simulink model "CompFeatures_testHarness"  (R2012b)
settings: Solver=FixedStepDiscrete  StartTime=0.0  StopTime=50  RelTol=1e-3
InitFcn:
  | N=256;
  | Fs = 1000;
  | bw = 5.6;
undefined symbols (not defined in the file): sigbuilder_block
libraries: simulink x4, ResultLoggerLib x3
settings Model: RequirementInfo={'other' '..\..\..\..\requirements\ebd_srs.doc' '@Simulink_requirement_item_4' 'true' 'Filter input signal via polyphase digital filter bank' 'Requirement' } %GIDa_bfa4a348_cd9f_4101_a776_3ea215f34dae  SldvGeneratedHarnessModel=TestUnitModel=CompFeatures|  RecordCoverage=on  CovMetricSettings=dcmtroie  CovHTMLOptions=-sRT=1 -aTS=1 -bRG=1 -bTC=0 -hTR=0 -nFC=0 -scm=1 -bcm=1 -xEv=0  CovExternalEMLEnable=on  Creator=aanantha  LastModifiedBy=klindqvi
settings DataIOCC: SaveFormat=Structure  SignalLoggingSaveFormat=ModelDataLogs  SaveOutput=off  SaveTime=off  SignalLoggingName=logsOut
settings OptimizationCC: InlineParams=on  OptimizeModelRefInitCode=on  LifeSpan=1
settings DebuggingCC: ReadBeforeWriteMsg=DisableAll  WriteAfterWriteMsg=DisableAll  WriteAfterReadMsg=DisableAll  SolverPrmCheckMsg=none  InheritedTsInSrcMsg=none  ParameterPrecisionLossMsg=none  FcnCallInpInsideContextMsg=EnableAllAsWarning  ModelReferenceSymbolNameMessage=none
settings HardwareCC: ProdLargestAtomicInteger=Long  ProdLargestAtomicFloat=Double  ProdEndianess=LittleEndian  ProdHWDeviceType=ARM Compatible->ARM Cortex
settings ModelReferenceCC: UpdateModelReferenceTargets=AssumeUpToDate  CheckModelReferenceTargetMessage=none
settings RTWCC: SystemTargetFile=ert.tlc  TemplateMakefile=ert_default_tmf  Description=Embedded Coder  GenerateReport=on  ProcessScript=ert_make_rtw_hook  IncludeHyperlinkInReport=on  LaunchReport=on  GenerateTraceInfo=on  GenerateTraceReportSl=on  GenerateTraceReportSf=on  GenerateTraceReportEml=on  GenerateCodeMetricsReport=on
settings CodeAppCC: IgnoreCustomStorageClasses=off
settings ERTTargetCC: CodeReplacementLibrary=GCC ARM Cortex-A8  MultiwordLength=2048  GenerateSampleERTMain=on  ERTCustomFileTemplate=example_file_process.tlc  ConvertIfToSwitch=off  SuppressUnreachableDefaultCases=off

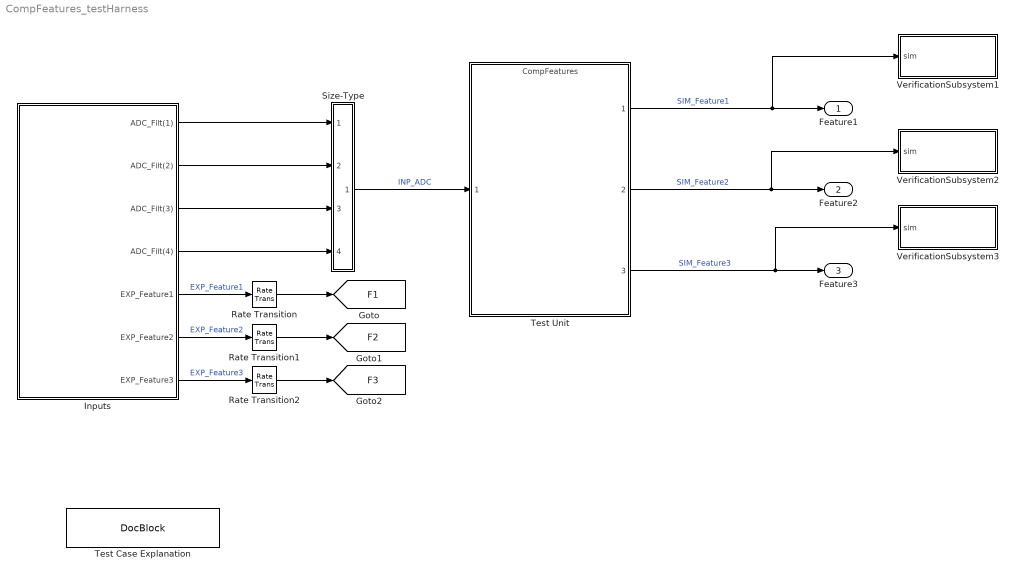
== system CompFeatures_testHarness ==
  Inputs : Subsystem  Tag=STV Subsys  RequirementInfo={'other' '..\..\..\..\requirements\ebd_srs.doc' '@REQ001- Filter input signal via polyphase digital filter bank' 'true' 'REQ001- Filter input signal via polyphase digital filter bank' '' } %GIDa_c0a67702_d4ee_4461_aee3_06328e90f161  LoadFcn=sigbuilder_block('load');  StartFcn=sigbuilder_block('start');  StopFcn=sigbuilder_block('stop');  ClipboardFcn=sigbuilder_block('clipboard');  mask(Sigbuilder block){}
      mask init:
      | if ~strcmp(get_param(bdroot(gcb),'SimulationStatus'),'stopped'),tuvar = sigbuilder_block('maskInit'); end
      settings: CopyFcn=sigbuilder_block('copy');  DeleteFcn=sigbuilder_block('delete');  ModelCloseFcn=sigbuilder_block('modelClose');  PreSaveFcn=sigbuilder_block('preSave');  PauseFcn=sigbuilder_block('pause');  ContinueFcn=sigbuilder_block('continue');  NameChangeFcn=sigbuilder_block('namechange');  OpenFcn=sigbuilder_block('open',[49.5 50.25 519.75 603 ]);  CloseFcn=sigbuilder_block('close');
      mask Display: plot(0, 0, 100, 100,[2, 2, 32, 32, 2], [68, 8, 8, 68, 68],[32, 2], [38, 38], [32, 19, 2],[53, 60, 44], [32, 17, 17, 2],[16, 16, 31, 31]);txt = getActiveGroup(gcbh);text(2, 100, txt,'verticalAlignment', 'top');
  Rate Transition : RateTransition  Integrity=off
  Rate Transition1 : RateTransition  Integrity=off
  Rate Transition2 : RateTransition  Integrity=off
  Size-Type : Subsystem
  Test Case Explanation : simulink/Model-Wide Utilities/DocBlock  DocumentType=Text
      content=|
      | Test case with default values because no SLDVDATA supplied
  Test Unit : ModelReference  ModelNameDialog=CompFeatures  SimulationMode=Normal  ModelReferenceVersion=1.280  CopyOfModelName=CompFeatures  DefaultDataLogging=on
  VerificationSubsystem1 : Subsystem
  VerificationSubsystem2 : Subsystem
  VerificationSubsystem3 : Subsystem
  Feature1 : Outport  OutDataTypeStr=single  PortDimensions=1  SampleTime=[0.08900000000000001,0]
  Feature2 : Outport  Port=2  OutDataTypeStr=single  PortDimensions=1  SampleTime=[0.08900000000000001,0]
  Feature3 : Outport  Port=3  OutDataTypeStr=single  PortDimensions=1  SampleTime=[0.08900000000000001,0]
  tag scope: F1=global, F2=global, F3=global
  wires:
  Size-Type/1(Out1) -> Test Unit/1  "INP_ADC"
  Test Unit/1 -> VerificationSubsystem1/1("sim "), Feature1/1  "SIM_Feature1"
  Test Unit/2 -> VerificationSubsystem2/1("sim "), Feature2/1  "SIM_Feature2"
  Test Unit/3 -> VerificationSubsystem3/1("sim "), Feature3/1  "SIM_Feature3"
  Inputs/5(EXP_Feature1) -> Rate Transition/1  "EXP_Feature1"
  Inputs/7(EXP_Feature3) -> Rate Transition2/1  "EXP_Feature3"
  Inputs/6(EXP_Feature2) -> Rate Transition1/1  "EXP_Feature2"
  Inputs/1(ADC_Filt(1)) -> Size-Type/1(In1)
  Inputs/2(ADC_Filt(2)) -> Size-Type/2(In2)
  Inputs/3(ADC_Filt(3)) -> Size-Type/3(In3)
  Inputs/4(ADC_Filt(4)) -> Size-Type/4(In4)
  Rate Transition/1 -> [F1]
  Rate Transition1/1 -> [F2]
  Rate Transition2/1 -> [F3]

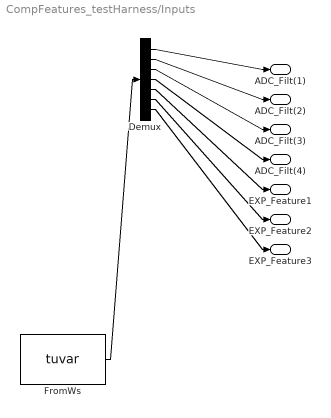
== system CompFeatures_testHarness/Inputs ==
  Demux : Demux  Tag=STV Demux  Outputs=7
  FromWs : FromWorkspace  Tag=STV FromWs  VariableName=tuvar  SampleTime=0
      SigBuilderData=|
      | dataSet(1).timeRange = [0 10]
      | dataSet(1).name = 'Test Case 1'
      | dataSet(2).timeRange = [0 10]
      | dataSet(2).name = 'Test Case 2'
      | sbobj.Name = 'Signal Builder'
      | sbobj.Groups(1).Name = 'Test Case 1'
      | sbobj.Groups(1).Signals(1).Name = 'ADC_Filt(1)'
      | sbobj.Groups(1).Signals(1).XData = [0 10]
      | sbobj.Groups(1).Signals(1).YData = [1 1]
      | sbobj.Groups(1).Signals(2).Name = 'ADC_Filt(2)'
      | sbobj.Groups(1).Signals(2).XData = [0 10]
      | sbobj.Groups(1).Signals(2).YData = [1 1]
      | sbobj.Groups(1).Signals(3).Name = 'ADC_Filt(3)'
      | sbobj.Groups(1).Signals(3).XData = [0 10]
      | sbobj.Groups(1).Signals(3).YData = [1 1]
      | sbobj.Groups(1).Signals(4).Name = 'ADC_Filt(4)'
      | sbobj.Groups(1).Signals(4).XData = [0 10]
      | sbobj.Groups(1).Signals(4).YData = [1 1]
      | sbobj.Groups(1).Signals(5).Name = 'EXP_Feature1'
      | sbobj.Groups(1).Signals(5).XData = [0 0.34 0.34 0.44 0.44 10]
      | sbobj.Groups(1).Signals(5).YData = [0 0 1.5 1.5 3 3]
      | sbobj.Groups(1).Signals(6).Name = 'EXP_Feature2'
      | sbobj.Groups(1).Signals(6).XData = [0 0.34 0.34 0.44 0.44 10]
      | sbobj.Groups(1).Signals(6).YData = [0 0 2 2 4 4]
      | sbobj.Groups(1).Signals(7).Name = 'EXP_Feature3'
      | sbobj.Groups(1).Signals(7).XData = [0 0.35 0.35 0.44 0.44 10]
      | sbobj.Groups(1).Signals(7).YData = [0 0 1.5 1.5 3 3]
      | sbobj.Groups(2).Name = 'Test Case 2'
      | sbobj.Groups(2).Signals(1).Name = 'ADC_Filt(1)'
      | sbobj.Groups(2).Signals(1).XData = [0 10]
      | sbobj.Groups(2).Signals(1).YData = [0 0]
      | sbobj.Groups(2).Signals(2).Name = 'ADC_Filt(2)'
      | sbobj.Groups(2).Signals(2).XData = [0 10]
      | sbobj.Groups(2).Signals(2).YData = [0 0]
      | sbobj.Groups(2).Signals(3).Name = 'ADC_Filt(3)'
      | sbobj.Groups(2).Signals(3).XData = [0 10]
      | sbobj.Groups(2).Signals(3).YData = [0 0]
      | sbobj.Groups(2).Signals(4).Name = 'ADC_Filt(4)'
      | sbobj.Groups(2).Signals(4).XData = [0 10]
      | sbobj.Groups(2).Signals(4).YData = [0 0]
      | sbobj.Groups(2).Signals(5).Name = 'EXP_Feature1'
      | sbobj.Groups(2).Signals(5).XData = [0 0.34 10]
      | sbobj.Groups(2).Signals(5).YData = [0 0 0]
      | sbobj.Groups(2).Signals(6).Name = 'EXP_Feature2'
      | sbobj.Groups(2).Signals(6).XData = [0 0.34 10]
      | sbobj.Groups(2).Signals(6).YData = [0 0 0]
      | sbobj.Groups(2).Signals(7).Name = 'EXP_Feature3'
      | sbobj.Groups(2).Signals(7).XData = [0 0.34 10]
      | sbobj.Groups(2).Signals(7).YData = [0 0 0]
  ADC_Filt(1) : Outport  Tag=STV Outport
  ADC_Filt(2) : Outport  Tag=STV Outport  Port=2
  ADC_Filt(3) : Outport  Tag=STV Outport  Port=3
  ADC_Filt(4) : Outport  Tag=STV Outport  Port=4
  EXP_Feature1 : Outport  Tag=STV Outport  Port=5
  EXP_Feature2 : Outport  Tag=STV Outport  Port=6
  EXP_Feature3 : Outport  Tag=STV Outport  Port=7
  wires:
  Demux/4 -> ADC_Filt(4)/1
  Demux/3 -> ADC_Filt(3)/1
  Demux/2 -> ADC_Filt(2)/1
  Demux/1 -> ADC_Filt(1)/1
  FromWs/1 -> Demux/1
  Demux/5 -> EXP_Feature1/1
  Demux/6 -> EXP_Feature2/1
  Demux/7 -> EXP_Feature3/1

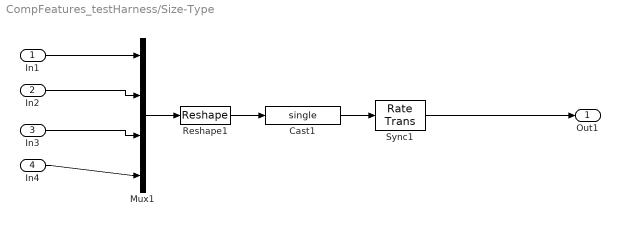
== system CompFeatures_testHarness/Size-Type ==
  In1 : Inport
  In2 : Inport  Port=2
  In3 : Inport  Port=3
  In4 : Inport  Port=4
  Cast1 : DataTypeConversion  OutDataTypeStr=single  SaturateOnIntegerOverflow=on  RndMeth=Zero
  Mux1 : Mux
  Reshape1 : Reshape  OutputDimensionality=Customize  OutputDimensions=4
  Sync1 : RateTransition  OutPortSampleTime=[0.08900000000000001,0]
  Out1 : Outport
  wires:
  Sync1/1 -> Out1/1
  Cast1/1 -> Sync1/1
  Reshape1/1 -> Cast1/1
  Mux1/1 -> Reshape1/1
  In4/1 -> Mux1/4
  In3/1 -> Mux1/3
  In2/1 -> Mux1/2
  In1/1 -> Mux1/1

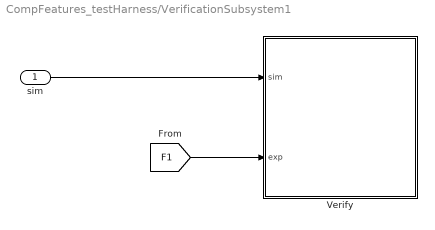
== system CompFeatures_testHarness/VerificationSubsystem1 ==
  "sim " : Inport
  Verify : Subsystem
  wires:
  "sim "/1 -> Verify/1(sim)
  [F1] -> Verify/2(exp)

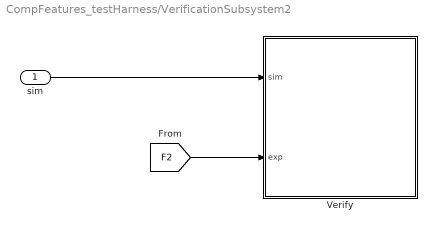
== system CompFeatures_testHarness/VerificationSubsystem2 ==
  "sim " : Inport
  Verify : Subsystem
  wires:
  [F2] -> Verify/2(exp)
  "sim "/1 -> Verify/1(sim)

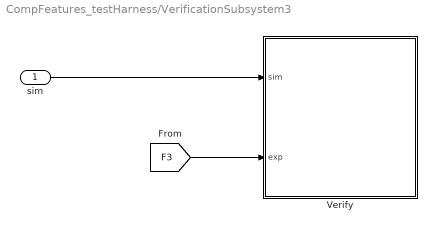
== system CompFeatures_testHarness/VerificationSubsystem3 ==
  "sim " : Inport
  Verify : Subsystem
  wires:
  "sim "/1 -> Verify/1(sim)
  [F3] -> Verify/2(exp)

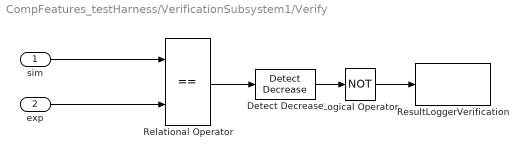
== system CompFeatures_testHarness/VerificationSubsystem1/Verify ==
  sim : Inport
  exp : Inport  Port=2
  Detect Decrease : simulink/Logic and Bit Operations/Detect Decrease  vinit=0.0  InputProcessing=Inherited  OutDataTypeStr=boolean
  Logical Operator : Logic  Operator=NOT  Inputs=1  AllPortsSameDT=off  OutDataTypeStr=boolean
  Relational Operator : RelationalOperator  Operator===  OutDataTypeStr=boolean
  ResultLoggerVerification : ResultLoggerLib/ResultLoggerVerification  Description=Verify the computation of feature 1  resultLoggerDescription=Verify the computation of feature 1
      settings: AttributesFormatString=%<Description>
  wires:
  sim/1 -> Relational Operator/1
  exp/1 -> Relational Operator/2
  Relational Operator/1 -> Detect Decrease/1
  Detect Decrease/1 -> Logical Operator/1
  Logical Operator/1 -> ResultLoggerVerification/1

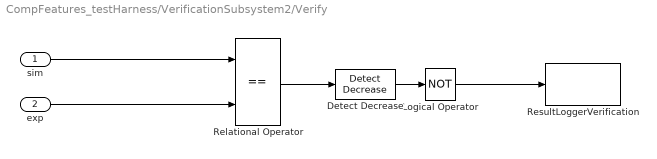
== system CompFeatures_testHarness/VerificationSubsystem2/Verify ==
  sim : Inport
  exp : Inport  Port=2
  Detect Decrease : simulink/Logic and Bit Operations/Detect Decrease  vinit=0.0  InputProcessing=Inherited  OutDataTypeStr=boolean
  Logical Operator : Logic  Operator=NOT  Inputs=1  AllPortsSameDT=off  OutDataTypeStr=boolean
  Relational Operator : RelationalOperator  Operator===  OutDataTypeStr=boolean
  ResultLoggerVerification : ResultLoggerLib/ResultLoggerVerification  Description=Verify the computation of feature 2  resultLoggerDescription=Verify the computation of feature 2
      settings: AttributesFormatString=%<Description>
  wires:
  Relational Operator/1 -> Detect Decrease/1
  exp/1 -> Relational Operator/2
  sim/1 -> Relational Operator/1
  Detect Decrease/1 -> Logical Operator/1
  Logical Operator/1 -> ResultLoggerVerification/1

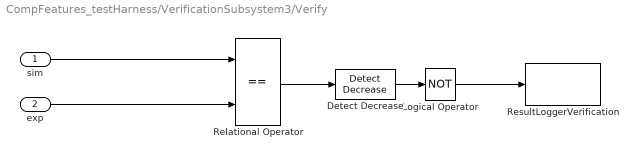
== system CompFeatures_testHarness/VerificationSubsystem3/Verify ==
  sim : Inport
  exp : Inport  Port=2
  Detect Decrease : simulink/Logic and Bit Operations/Detect Decrease  vinit=0.0  InputProcessing=Inherited  OutDataTypeStr=boolean
  Logical Operator : Logic  Operator=NOT  Inputs=1  AllPortsSameDT=off  OutDataTypeStr=boolean
  Relational Operator : RelationalOperator  Operator===  OutDataTypeStr=boolean
  ResultLoggerVerification : ResultLoggerLib/ResultLoggerVerification  Description=Verify the computation of feature 3  resultLoggerDescription=Verify the computation of feature 3
      settings: AttributesFormatString=%<Description>
  wires:
  sim/1 -> Relational Operator/1
  exp/1 -> Relational Operator/2
  Relational Operator/1 -> Detect Decrease/1
  Detect Decrease/1 -> Logical Operator/1
  Logical Operator/1 -> ResultLoggerVerification/1
